simulink model "caracterizacion"  (Simulink 8.0)
settings: Solver=ode5  StartTime=0.0  StopTime=inf  RelTol=1e-3
undefined symbols (not defined in the file or in its folder): National_Instruments, PCI
libraries: rtwinlib x2, simulink x1
settings Model: Creator=oscar_mau.fernandez  LastModifiedBy=HenryPareja  SimulationMode=external
settings DataIOCC: SignalLoggingSaveFormat=ModelDataLogs
settings DebuggingCC: FcnCallInpInsideContextMsg=EnableAllAsWarning
settings HardwareCC: ProdIntDivRoundTo=Zero  ProdEndianess=LittleEndian  ProdHWDeviceType=Generic->32-bit x86 compatible
settings RTWCC: SystemTargetFile=rtwin.tlc  TemplateMakefile=rtwin.tmf  Description=Real-Time Windows Target  RetainRTWFile=on  ProcessScript=rtwin_make_rtw_hook  RTWCompilerOptimization=On
settings CodeAppCC: MaxIdLength=95
settings RTWinTargetCC: TargetLibSuffix=_rtwin.lib  TargetPreCompLibLocation=C:\Program Files\MATLAB\R2012b\toolbox\rtw\targets\rtwin\lib\win64  CodeReplacementLibrary=ANSI_C  RTWinDir=C:/PROGRA~1/MATLAB/R2012b/toolbox/rtw/targets/rtwin  TargetArch=win64  RebuildAll=on

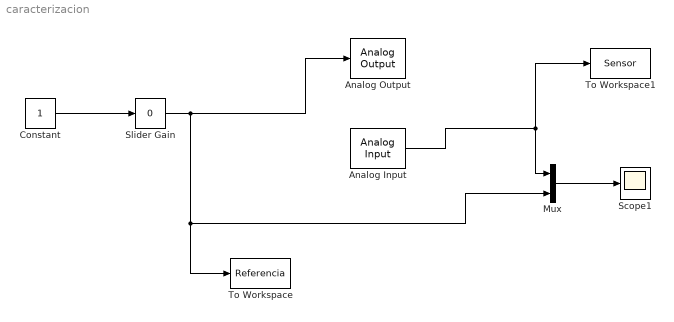
== system caracterizacion ==
  Analog Input : rtwinlib/Analog Input  SampleTime=0.01  MaxMissedTicks=10  ShowMissedTicks=off  YieldWhenWaiting=off  DrvName=National_Instruments/PCI-6221  DrvAddress=4294967295  DrvOptions=[1 0 0 0 0]  Channels=1  RangeMode=1  VoltRange=2  DataType=1
      settings: AttributesFormatString=National Instruments\nPCI-6221 [auto]
  Analog Output : rtwinlib/Analog Output  SampleTime=0.01  MaxMissedTicks=10  ShowMissedTicks=off  YieldWhenWaiting=off  DrvName=National_Instruments/PCI-6221  DrvAddress=4294967295  DrvOptions=[1 0 0 0 0]  Channels=1  RangeMode=1  VoltRange=1  InitialValue=0  FinalValue=5
      settings: AttributesFormatString=National Instruments\nPCI-6221 [auto]
  Constant : Constant
  Mux : Mux  Inputs=2
  Scope1 : Scope
      settings: TimeRange=100  YMin=0  YMax=4.5
  Slider Gain : simulink/Math Operations/Slider Gain  low=0  gain=0  high=5
  To Workspace : ToWorkspace  VariableName=Referencia  SampleTime=0.01
  To Workspace1 : ToWorkspace  VariableName=Sensor  SampleTime=0.01
  wires:
  Analog Input/1 -> Mux/1, To Workspace1/1
  Mux/1 -> Scope1/1
  Slider Gain/1 -> To Workspace/1, Mux/2, Analog Output/1
  Constant/1 -> Slider Gain/1
